simulink model "samerHARDWAREPOTread"  (R2025b)
settings: Solver=FixedStepDiscrete  StartTime=0.0  StopTime=inf  RelTol=1e-3  EnableMultiTasking=on
libraries: arduinolib x18, slpidlib x6, simulink x2
settings Model: ExtModeTrigDuration=2  Creator=Ahmed Sedky  LastModifiedBy=Samer FARAJ
settings OptimizationCC: EnhancedBackFolding=on  PassReuseOutputArgsAs=Individual arguments  ZeroExternalMemoryAtStartup=off  ZeroInternalMemoryAtStartup=off  MaxStackSize=64  OptimizeBlockOrder=speed  DifferentSizesBufferReuse=on  OptimizationCustomize=off  EfficientTunableParamExpr=on
settings DebuggingCC: ParameterTunabilityLossMsg=error
settings HardwareCC: ProdBitPerInt=16.0  ProdBitPerPointer=16.0  ProdBitPerSizeT=16.0  ProdBitPerPtrDiffT=16.0  ProdLargestAtomicFloat=None  ProdWordSize=8.0  ProdHWDeviceType=Atmel->AVR
settings SFSimCC: MATLABDynamicMemAlloc=off
settings RTWCC: SystemTargetFile=ert.tlc  HardwareBoard=Arduino Mega 2560  TemplateMakefile=ert_default_tmf  Toolchain=Arduino AVR  BuildConfiguration=Faster Runs  GPUComputeCapability=3.5  Description=Embedded Coder
settings CodeAppCC: ForceParamTrailComments=on  IgnoreCustomStorageClasses=off  OperatorAnnotations=on  SimulinkDataObjDesc=on  SFDataObjDesc=on  InsertBlockDesc=on
settings ERTTargetCC: ExtModeTransport=3.0  ExtModeStaticAlloc=on  ExtModeAutomaticAllocSize=off  ExtModeStaticAllocSize=2048.0  ExtModeMexFile=ext_xcp  ExtModeIntrfLevel=Level2 - Open  InlinedParameterPlacement=Hierarchical  DynamicArrayContainerType=coder::array  SupportContinuousTime=on  SupportVariableSizeSignals=on

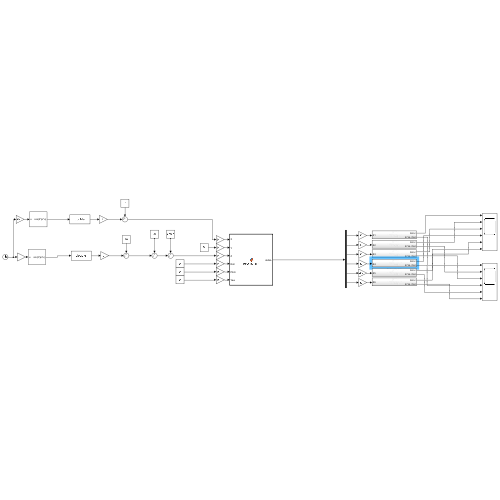
[thumbnail: Simulink's stored preview of the top-level diagram]
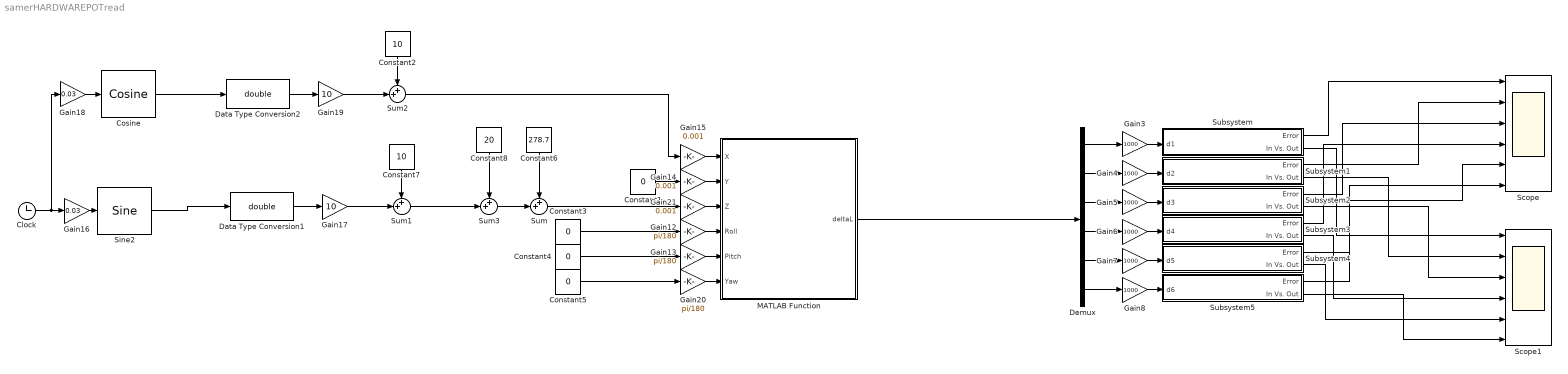
== system samerHARDWAREPOTread ==
  Clock : Clock
  Constant{1,3..5} (4 alike) : Constant  Value=0
  Constant2 : Constant  Value=10
  Constant6 : Constant  Value=278.7
  Constant7 : Constant  Value=10
  Constant8 : Constant  Value=20
  Cosine : simulink/Lookup Tables/Cosine  Formula=cos(2*pi*u)  NumDataPoints=(2^5)+1  OutputWordLength=16  InternalRulePriority=Speed
  Data Type Conversion1 : DataTypeConversion  OutDataTypeStr=double  SaturateOnIntegerOverflow=off  RndMeth=Floor
  Data Type Conversion2 : DataTypeConversion  OutDataTypeStr=double  SaturateOnIntegerOverflow=off  RndMeth=Floor
  Demux : Demux  Outputs=6
  Gain12 : Gain  Gain=pi/180
  Gain13 : Gain  Gain=pi/180
  Gain14 : Gain  Gain=0.001
  Gain15 : Gain  Gain=0.001
  Gain16 : Gain  Gain=0.03
  Gain17 : Gain  Gain=10
  Gain18 : Gain  Gain=0.03
  Gain19 : Gain  Gain=10
  Gain20 : Gain  Gain=pi/180
  Gain21 : Gain  Gain=0.001
  Gain{3..8} (6 alike) : Gain  Gain=1000
  MATLAB Function : MATLAB Function  TreatAsAtomicUnit=on
  Scope : Scope  NumInputPorts=6
      settings: ActiveDisplayYMinimum=15.51881  ActiveDisplayYMaximum=26.12546
  Scope1 : Scope  NumInputPorts=6
      settings: ActiveDisplayYMinimum=-3.1331  ActiveDisplayYMaximum=28.1979  DataLoggingVariableName=ScopeData2
  Sine2 : simulink/Lookup Tables/Sine  Formula=sin(2*pi*u)  NumDataPoints=(2^5)+1  OutputWordLength=16  InternalRulePriority=Speed
  Subsystem : Subsystem
  Subsystem1 : Subsystem
  Subsystem2 : Subsystem
  Subsystem3 : Subsystem
  Subsystem4 : Subsystem
  Subsystem5 : Subsystem
  Sum{,1..3} (4 alike) : Sum  Inputs=++|
  wires:
  Demux/1 -> Gain3/1
  Demux/6 -> Gain8/1
  Demux/3 -> Gain5/1
  Demux/4 -> Gain6/1
  Demux/5 -> Gain7/1
  Demux/2 -> Gain4/1
  Gain3/1 -> Subsystem/1(d1)
  Gain4/1 -> Subsystem1/1(d2)
  Gain5/1 -> Subsystem2/1(d3)
  Gain6/1 -> Subsystem3/1(d4)
  Gain7/1 -> Subsystem4/1(d5)
  Gain8/1 -> Subsystem5/1(d6)
  Subsystem/1(Error) -> Scope/1
  Subsystem1/1(Error) -> Scope/2
  Subsystem2/1(Error) -> Scope/3
  Subsystem3/1(Error) -> Scope/4
  Subsystem4/1(Error) -> Scope/5
  Subsystem5/1(Error) -> Scope/6
  Subsystem/2(In Vs. Out) -> Scope1/1
  Subsystem1/2(In Vs. Out) -> Scope1/2
  Subsystem2/2(In Vs. Out) -> Scope1/3
  Subsystem3/2(In Vs. Out) -> Scope1/4
  Subsystem4/2(In Vs. Out) -> Scope1/5
  Subsystem5/2(In Vs. Out) -> Scope1/6
  Constant8/1 -> Sum3/1
  Gain21/1 -> MATLAB Function/3(Z)
  Gain18/1 -> Cosine/1
  Gain15/1 -> MATLAB Function/1(X)
  Sum3/1 -> Sum/2
  Gain16/1 -> Sine2/1
  Cosine/1 -> Data Type Conversion2/1
  Gain20/1 -> MATLAB Function/6(Yaw)
  Gain19/1 -> Sum2/2
  Gain17/1 -> Sum1/2
  Data Type Conversion2/1 -> Gain19/1
  Constant6/1 -> Sum/1
  Sine2/1 -> Data Type Conversion1/1
  Constant7/1 -> Sum1/1
  Constant3/1 -> Gain12/1
  Clock/1 -> Gain16/1, Gain18/1
  Constant2/1 -> Sum2/1
  Sum/1 -> Gain21/1
  Gain14/1 -> MATLAB Function/2(Y)
  Constant1/1 -> Gain14/1
  Constant5/1 -> Gain20/1
  Sum1/1 -> Sum3/2
  Sum2/1 -> Gain15/1
  Constant4/1 -> Gain13/1
  Gain12/1 -> MATLAB Function/4(Roll)
  Data Type Conversion1/1 -> Gain17/1
  Gain13/1 -> MATLAB Function/5(Pitch)
  MATLAB Function/1(deltaL) -> Demux/1

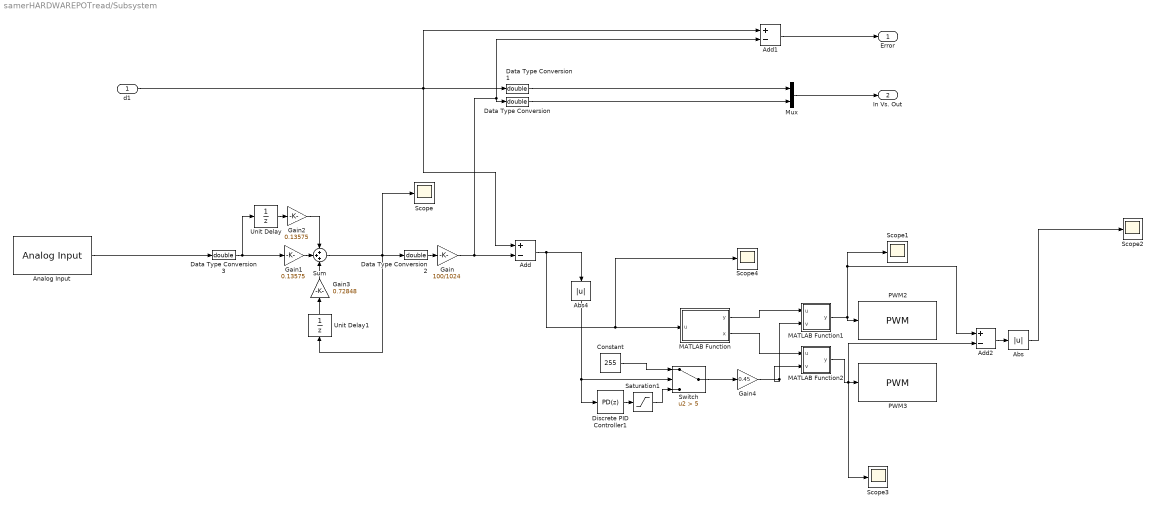
== system samerHARDWAREPOTread/Subsystem ==
  d1 : Inport
  Abs : Abs  SaturateOnIntegerOverflow=off
  Abs4 : Abs  SaturateOnIntegerOverflow=off
  Add : Sum  Inputs=+-
  Add1 : Sum  Inputs=+-
  Add2 : Sum  Inputs=+-
  Analog Input : arduinolib/Analog Input  pinNumber=0  ReadResultsOnly=off  ConversionTriggerSource=Software  ExternalTriggerType=uint32( 0 )  OutputDataType=uint16  EnableConversionCompleteNotify=off  EnableOuputStatus=off  SampleTime=0.01  blockPlatform=arduino
  Constant : Constant  Value=255
  Data Type Conversion{,1..3} (4 alike) : DataTypeConversion  OutDataTypeStr=double  SaturateOnIntegerOverflow=off  RndMeth=Floor
  Discrete PID Controller1 : slpidlib/PID Controller  Controller=PD  Form=Parallel  TimeDomain=Discrete-time  UseExternalTs=off  SampleTime=0.01  IntegratorMethod=Forward Euler  FilterMethod=Forward Euler  ControllerParametersSource=internal  P=325  I=3  UseKiTs=off  D=.75  UseExternalDerivativeSource=off  N=1  UseFilter=off  TunerSelectOption=Transfer Function Based (PID Tuner App)  InitialConditionSource=internal  InitialConditionForIntegrator=0  InitialConditionForFilter=0  DifferentiatorICPrevScaledInput=0  ExternalReset=none  TrackingMode=off  Kt=1  LimitOutput=off  SatLimitsSource=internal  UpperSaturationLimit=inf  LowerSaturationLimit=-inf  LinearizeAsGain=off  AntiWindupMode=none  Kb=1  LimitIntegrator=off  UpperIntegratorSaturationLimit=inf  LowerIntegratorSaturationLimit=-inf  POutMin=[]  POutMax=[]  IOutMin=[]  IOutMax=[]  DOutMin=[]  DOutMax=[]  NOutMin=[]  NOutMax=[]  SumOutMin=[]  SumOutMax=[]  SaturationOutMin=[]  SaturationOutMax=[]  PParamMin=[]  PParamMax=[]  IParamMin=[]  IParamMax=[]  DParamMin=[]  DParamMax=[]  NParamMin=[]  NParamMax=[]  KbParamMin=[]  KbParamMax=[]  KtParamMin=[]  KtParamMax=[]  KbOutMin=[]  KbOutMax=[]  KtOutMin=[]  KtOutMax=[]  IntegratorOutMin=[]  IntegratorOutMax=[]  FilterOutMin=[]  FilterOutMax=[]  SumI1OutMin=[]  SumI1OutMax=[]  SumI2OutMin=[]  SumI2OutMax=[]  SumI3OutMin=[]  SumI3OutMax=[]  SumI4OutMin=[]  SumI4OutMax=[]  SumDOutMin=[]  SumDOutMax=[]  DifferentiatorOutMin=[]  DifferentiatorOutMax=[]  FilterDiffOutCoefMin=[]  FilterDiffOutCoefMax=[]  ReciprocalOutMin=[]  ReciprocalOutMax=[]  SumDenOutMin=[]  SumDenOutMax=[]  SumNumOutMin=[]  SumNumOutMax=[]  DivideOutMin=[]  DivideOutMax=[]  UdiffTsProdOutMin=[]  UdiffTsProdOutMax=[]  NTsProdOutMin=[]  NTsProdOutMax=[]  UintegralTsProdOutMin=[]  UintegralTsProdOutMax=[]  UngainTsProdOutMin=[]  UngainTsProdOutMax=[]  ClampingZeroOutDataTypeStr=Inherit: Inherit via back propagation  ClampingZeroOutMin=[]  ClampingZeroOutMax=[]  FilterDenConstantOutDataTypeStr=Inherit: Inherit via back propagation  FilterDenConstantOutMin=[]  FilterDenConstantOutMax=[]  PCopyOutDataTypeStr=Inherit: Inherit via back propagation  PCopyOutMin=[]  PCopyOutMax=[]  NCopyOutDataTypeStr=Inherit: Inherit via back propagation  NCopyOutMin=[]  NCopyOutMax=[]  IntegratorContinuousStateAttributes=''  IntegratorStateMustResolveToSignalObject=off  IntegratorRTWStateStorageClass=Auto  FilterContinuousStateAttributes=''  FilterStateMustResolveToSignalObject=off  FilterRTWStateStorageClass=Auto  ParallelPVariant=InternalParameters  IdealPVariant=Disabled  IVariant=Disabled  DVariant=InternalParameters  IntegratorVariant=Disabled  SatVariant=Disabled  AWVariant=Disabled  PCopyVariant=Disabled  TRVariant=Disabled  FdbkBlocksVariant=Forward  IdealPFdbkVariant=Disabled  SatFdbkVariant=Disabled  DerivativeFilterVariant=Differentiator  NVariant=Passthrough  NCopyVariant=Disabled_SignalSpec  FilterICVariant=InternalICsDifferentiator  IntegratorICVariant=Disabled  ExternalResetVariant=Disabled  TRSumVariant=Passthrough  SumFdbkVariant=Disabled  SumVariant=Sum_PD  TsampFilterVariant=InternalTs  TsampNgainVariant=Passthrough  TsampIntegralVariant=Disabled_SignalSpec  ExternalSaturationOutDataTypeStr=Inherit: Same as second input  DerivativeSourceVariant=ErrorSignal  PreIntVariant=InternalPreInt
      settings: LibrarySourceBlock=simulink/Discrete/Discrete PID Controller
  Gain : Gain  Gain=100/1024
  Gain1 : Gain  Gain=0.13575
  Gain2 : Gain  Gain=0.13575
  Gain3 : Gain  Gain=0.72848
  Gain4 : Gain  Gain=0.45
  MATLAB Function : MATLAB Function  TreatAsAtomicUnit=on
  MATLAB Function1 : MATLAB Function  TreatAsAtomicUnit=on
  MATLAB Function2 : MATLAB Function  TreatAsAtomicUnit=on
  Mux : Mux  Inputs=2
  PWM2 : arduinolib/PWM  pinNumber=2  frequencyType=Default  desiredFrequency=490.2  achievableFrequency=490.2
  PWM3 : arduinolib/PWM  pinNumber=3  frequencyType=Default  desiredFrequency=490.2  achievableFrequency=490.2
  Saturation1 : Saturate  UpperLimit=200  LowerLimit=0
  Scope{,1..4} (5 alike) : Scope
      Scope settings: ActiveDisplayYMinimum=-89.3058  ActiveDisplayYMaximum=803.75221
      Scope1 settings: ActiveDisplayYMinimum=-31.875  ActiveDisplayYMaximum=286.875  DataLoggingVariableName=ScopeData2
      Scope2 settings: DataLoggingVariableName=ScopeData3
      Scope3 settings: ActiveDisplayYMinimum=-31.875  ActiveDisplayYMaximum=286.875  DataLoggingVariableName=ScopeData4
      Scope4 settings: ActiveDisplayYMinimum=-38.33565  ActiveDisplayYMaximum=48.7182
  Sum : Sum  Inputs=+++
  Switch : Switch  Criteria=u2 > Threshold  Threshold=5  SaturateOnIntegerOverflow=off  InputSameDT=off
  Unit Delay : UnitDelay  SampleTime=-1  HasFrameUpgradeWarning=on
  Unit Delay1 : UnitDelay  SampleTime=-1  HasFrameUpgradeWarning=on
  Error : Outport
  In Vs. Out : Outport  Port=2
  wires:
  Unit Delay/1 -> Gain2/1
  Gain3/1 -> Sum/3
  Add2/1 -> Abs/1
  MATLAB Function1/1(y) -> PWM2/1, Add2/1, Scope1/1
  Data Type Conversion2/1 -> Gain/1
  Abs/1 -> Scope2/1
  MATLAB Function2/1(y) -> Scope3/1, Add2/2, PWM3/1
  Add/1 -> Abs4/1, Scope4/1, MATLAB Function/1(u)
  Saturation1/1 -> Switch/3
  Analog Input/1 -> Data Type Conversion3/1
  Unit Delay1/1 -> Gain3/1
  Gain/1 -> Data Type Conversion/1, Add1/2, Add/2
  d1/1 -> Data Type Conversion1/1, Add1/1, Add/1
  Discrete PID Controller1/1 -> Saturation1/1
  Constant/1 -> Switch/1
  Data Type Conversion/1 -> Mux/2
  Data Type Conversion1/1 -> Mux/1
  Mux/1 -> In Vs. Out/1
  Data Type Conversion3/1 -> Unit Delay/1, Gain1/1
  Sum/1 -> Scope/1, Data Type Conversion2/1, Unit Delay1/1
  Abs4/1 -> Discrete PID Controller1/1, Switch/2
  Switch/1 -> Gain4/1
  Gain4/1 -> MATLAB Function2/2(v), MATLAB Function1/2(v)
  MATLAB Function/1(y) -> MATLAB Function1/1(u)
  MATLAB Function/2(x) -> MATLAB Function2/1(u)
  Gain1/1 -> Sum/2
  Gain2/1 -> Sum/1
  Add1/1 -> Error/1

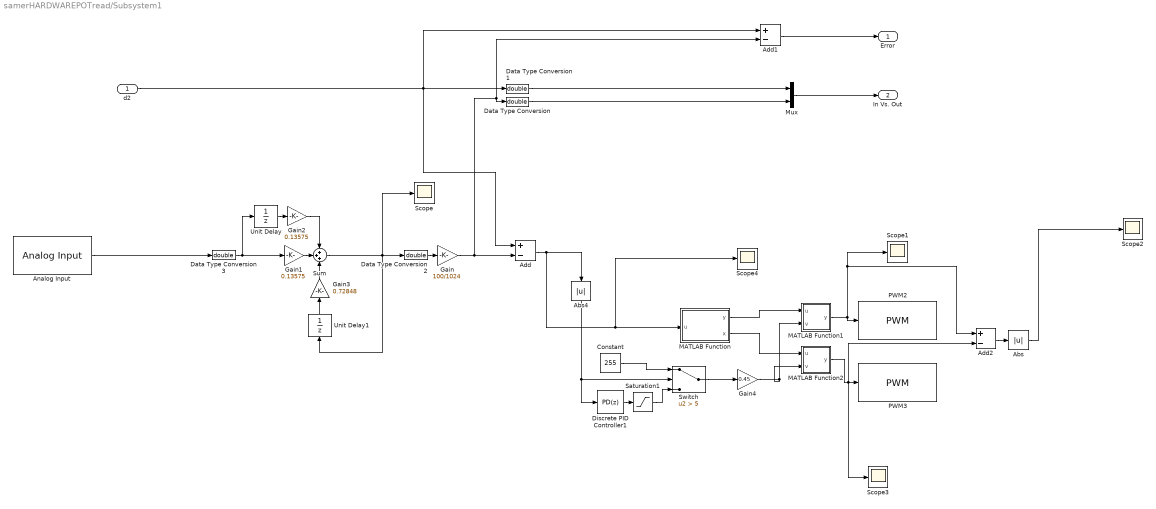
== system samerHARDWAREPOTread/Subsystem1 ==
  d2 : Inport
  Abs : Abs  SaturateOnIntegerOverflow=off
  Abs4 : Abs  SaturateOnIntegerOverflow=off
  Add : Sum  Inputs=+-
  Add1 : Sum  Inputs=+-
  Add2 : Sum  Inputs=+-
  Analog Input : arduinolib/Analog Input  pinNumber=5  ReadResultsOnly=off  ConversionTriggerSource=Software  ExternalTriggerType=uint32( 0 )  OutputDataType=uint16  EnableConversionCompleteNotify=off  EnableOuputStatus=off  SampleTime=0.01  blockPlatform=arduino
  Constant : Constant  Value=255
  Data Type Conversion{,1..3} (4 alike) : DataTypeConversion  OutDataTypeStr=double  SaturateOnIntegerOverflow=off  RndMeth=Floor
  Discrete PID Controller1 : slpidlib/PID Controller  Controller=PD  Form=Parallel  TimeDomain=Discrete-time  UseExternalTs=off  SampleTime=0.01  IntegratorMethod=Forward Euler  FilterMethod=Forward Euler  ControllerParametersSource=internal  P=325  I=3  UseKiTs=off  D=.75  N=1  UseFilter=off  TunerSelectOption=Transfer Function Based (PID Tuner App)  InitialConditionSource=internal  InitialConditionForIntegrator=0  InitialConditionForFilter=0  DifferentiatorICPrevScaledInput=0  ExternalReset=none  TrackingMode=off  Kt=1  LimitOutput=off  SatLimitsSource=internal  UpperSaturationLimit=inf  LowerSaturationLimit=-inf  LinearizeAsGain=off  AntiWindupMode=none  Kb=1  LimitIntegrator=off  UpperIntegratorSaturationLimit=inf  LowerIntegratorSaturationLimit=-inf  POutMin=[]  POutMax=[]  IOutMin=[]  IOutMax=[]  DOutMin=[]  DOutMax=[]  NOutMin=[]  NOutMax=[]  SumOutMin=[]  SumOutMax=[]  SaturationOutMin=[]  SaturationOutMax=[]  PParamMin=[]  PParamMax=[]  IParamMin=[]  IParamMax=[]  DParamMin=[]  DParamMax=[]  NParamMin=[]  NParamMax=[]  KbParamMin=[]  KbParamMax=[]  KtParamMin=[]  KtParamMax=[]  KbOutMin=[]  KbOutMax=[]  KtOutMin=[]  KtOutMax=[]  IntegratorOutMin=[]  IntegratorOutMax=[]  FilterOutMin=[]  FilterOutMax=[]  SumI1OutMin=[]  SumI1OutMax=[]  SumI2OutMin=[]  SumI2OutMax=[]  SumI3OutMin=[]  SumI3OutMax=[]  SumI4OutMin=[]  SumI4OutMax=[]  SumDOutMin=[]  SumDOutMax=[]  DifferentiatorOutMin=[]  DifferentiatorOutMax=[]  FilterDiffOutCoefMin=[]  FilterDiffOutCoefMax=[]  ReciprocalOutMin=[]  ReciprocalOutMax=[]  SumDenOutMin=[]  SumDenOutMax=[]  SumNumOutMin=[]  SumNumOutMax=[]  DivideOutMin=[]  DivideOutMax=[]  UdiffTsProdOutMin=[]  UdiffTsProdOutMax=[]  NTsProdOutMin=[]  NTsProdOutMax=[]  UintegralTsProdOutMin=[]  UintegralTsProdOutMax=[]  UngainTsProdOutMin=[]  UngainTsProdOutMax=[]  ClampingZeroOutDataTypeStr=Inherit: Inherit via back propagation  ClampingZeroOutMin=[]  ClampingZeroOutMax=[]  FilterDenConstantOutDataTypeStr=Inherit: Inherit via back propagation  FilterDenConstantOutMin=[]  FilterDenConstantOutMax=[]  PCopyOutDataTypeStr=Inherit: Inherit via back propagation  PCopyOutMin=[]  PCopyOutMax=[]  NCopyOutDataTypeStr=Inherit: Inherit via back propagation  NCopyOutMin=[]  NCopyOutMax=[]  IntegratorContinuousStateAttributes=''  IntegratorStateMustResolveToSignalObject=off  IntegratorRTWStateStorageClass=Auto  FilterContinuousStateAttributes=''  FilterStateMustResolveToSignalObject=off  FilterRTWStateStorageClass=Auto  ParallelPVariant=InternalParameters  IdealPVariant=Disabled  IVariant=Disabled  DVariant=InternalParameters  IntegratorVariant=Disabled  SatVariant=Disabled  AWVariant=Disabled  PCopyVariant=Disabled  TRVariant=Disabled  FdbkBlocksVariant=Forward  IdealPFdbkVariant=Disabled  SatFdbkVariant=Disabled  DerivativeFilterVariant=Differentiator  NVariant=Passthrough  NCopyVariant=Disabled_SignalSpec  FilterICVariant=InternalICsDifferentiator  IntegratorICVariant=Disabled  ExternalResetVariant=Disabled  TRSumVariant=Passthrough  SumFdbkVariant=Disabled  SumVariant=Sum_PD  TsampFilterVariant=InternalTs  TsampNgainVariant=Passthrough  TsampIntegralVariant=Disabled_SignalSpec  ExternalSaturationOutDataTypeStr=Inherit: Same as second input
      settings: LibrarySourceBlock=simulink/Discrete/Discrete PID Controller
  Gain : Gain  Gain=100/1024
  Gain1 : Gain  Gain=0.13575
  Gain2 : Gain  Gain=0.13575
  Gain3 : Gain  Gain=0.72848
  Gain4 : Gain  Gain=0.45
  MATLAB Function : MATLAB Function  TreatAsAtomicUnit=on
  MATLAB Function1 : MATLAB Function  TreatAsAtomicUnit=on
  MATLAB Function2 : MATLAB Function  TreatAsAtomicUnit=on
  Mux : Mux  Inputs=2
  PWM2 : arduinolib/PWM  pinNumber=4  frequencyType=Default  desiredFrequency=490.2  achievableFrequency=490.2
  PWM3 : arduinolib/PWM  pinNumber=5  frequencyType=Default  desiredFrequency=490.2  achievableFrequency=490.2
  Saturation1 : Saturate  UpperLimit=200  LowerLimit=0
  Scope{,1..4} (5 alike) : Scope
      Scope settings: ActiveDisplayYMinimum=-89.3058  ActiveDisplayYMaximum=803.75221
      Scope1 settings: ActiveDisplayYMinimum=-31.875  ActiveDisplayYMaximum=286.875  DataLoggingVariableName=ScopeData2
      Scope2 settings: DataLoggingVariableName=ScopeData3
      Scope3 settings: ActiveDisplayYMinimum=-31.875  ActiveDisplayYMaximum=286.875  DataLoggingVariableName=ScopeData4
      Scope4 settings: ActiveDisplayYMinimum=-38.33565  ActiveDisplayYMaximum=48.7182
  Sum : Sum  Inputs=+++
  Switch : Switch  Criteria=u2 > Threshold  Threshold=5  SaturateOnIntegerOverflow=off  InputSameDT=off
  Unit Delay : UnitDelay  SampleTime=-1  HasFrameUpgradeWarning=on
  Unit Delay1 : UnitDelay  SampleTime=-1  HasFrameUpgradeWarning=on
  Error : Outport
  In Vs. Out : Outport  Port=2
  wires:
  Unit Delay/1 -> Gain2/1
  Gain3/1 -> Sum/3
  Add2/1 -> Abs/1
  MATLAB Function1/1(y) -> PWM2/1, Add2/1, Scope1/1
  Data Type Conversion2/1 -> Gain/1
  Abs/1 -> Scope2/1
  MATLAB Function2/1(y) -> Scope3/1, Add2/2, PWM3/1
  Add/1 -> Abs4/1, Scope4/1, MATLAB Function/1(u)
  Saturation1/1 -> Switch/3
  Analog Input/1 -> Data Type Conversion3/1
  Unit Delay1/1 -> Gain3/1
  Gain/1 -> Data Type Conversion/1, Add1/2, Add/2
  d2/1 -> Data Type Conversion1/1, Add1/1, Add/1
  Discrete PID Controller1/1 -> Saturation1/1
  Constant/1 -> Switch/1
  Data Type Conversion/1 -> Mux/2
  Data Type Conversion1/1 -> Mux/1
  Mux/1 -> In Vs. Out/1
  Data Type Conversion3/1 -> Unit Delay/1, Gain1/1
  Sum/1 -> Scope/1, Data Type Conversion2/1, Unit Delay1/1
  Abs4/1 -> Discrete PID Controller1/1, Switch/2
  Switch/1 -> Gain4/1
  Gain4/1 -> MATLAB Function2/2(v), MATLAB Function1/2(v)
  MATLAB Function/1(y) -> MATLAB Function1/1(u)
  MATLAB Function/2(x) -> MATLAB Function2/1(u)
  Gain1/1 -> Sum/2
  Gain2/1 -> Sum/1
  Add1/1 -> Error/1

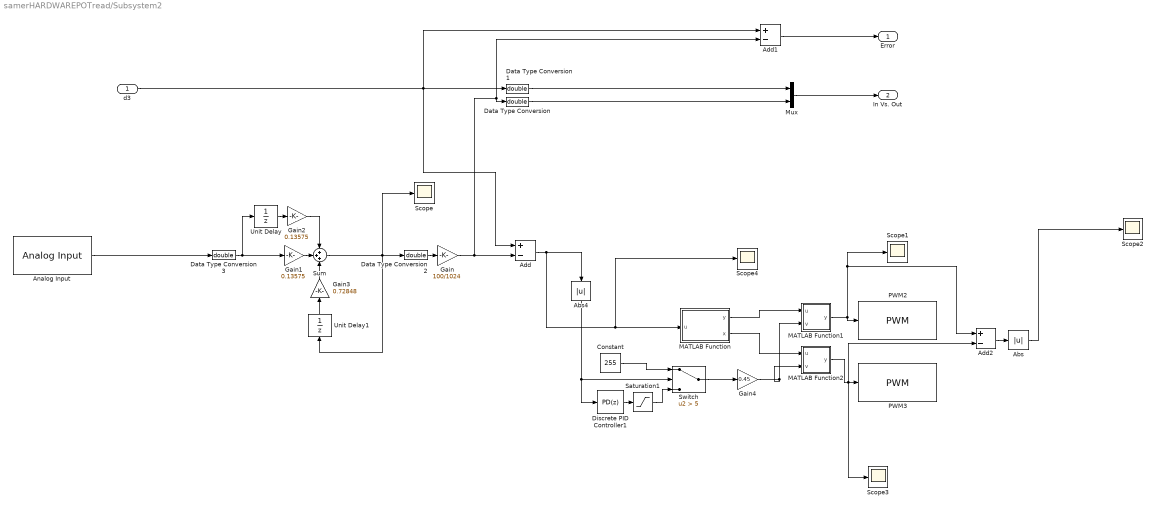
== system samerHARDWAREPOTread/Subsystem2 ==
  d3 : Inport
  Abs : Abs  SaturateOnIntegerOverflow=off
  Abs4 : Abs  SaturateOnIntegerOverflow=off
  Add : Sum  Inputs=+-
  Add1 : Sum  Inputs=+-
  Add2 : Sum  Inputs=+-
  Analog Input : arduinolib/Analog Input  pinNumber=4  ReadResultsOnly=off  ConversionTriggerSource=Software  ExternalTriggerType=uint32( 0 )  OutputDataType=uint16  EnableConversionCompleteNotify=off  EnableOuputStatus=off  SampleTime=0.01  blockPlatform=arduino
  Constant : Constant  Value=255
  Data Type Conversion{,1..3} (4 alike) : DataTypeConversion  OutDataTypeStr=double  SaturateOnIntegerOverflow=off  RndMeth=Floor
  Discrete PID Controller1 : slpidlib/PID Controller  Controller=PD  Form=Parallel  TimeDomain=Discrete-time  UseExternalTs=off  SampleTime=0.01  IntegratorMethod=Forward Euler  FilterMethod=Forward Euler  ControllerParametersSource=internal  P=325  I=3  UseKiTs=off  D=.75  UseExternalDerivativeSource=off  N=1  UseFilter=off  TunerSelectOption=Transfer Function Based (PID Tuner App)  InitialConditionSource=internal  InitialConditionForIntegrator=0  InitialConditionForFilter=0  DifferentiatorICPrevScaledInput=0  ExternalReset=none  TrackingMode=off  Kt=1  LimitOutput=off  SatLimitsSource=internal  UpperSaturationLimit=inf  LowerSaturationLimit=-inf  LinearizeAsGain=off  AntiWindupMode=none  Kb=1  LimitIntegrator=off  UpperIntegratorSaturationLimit=inf  LowerIntegratorSaturationLimit=-inf  POutMin=[]  POutMax=[]  IOutMin=[]  IOutMax=[]  DOutMin=[]  DOutMax=[]  NOutMin=[]  NOutMax=[]  SumOutMin=[]  SumOutMax=[]  SaturationOutMin=[]  SaturationOutMax=[]  PParamMin=[]  PParamMax=[]  IParamMin=[]  IParamMax=[]  DParamMin=[]  DParamMax=[]  NParamMin=[]  NParamMax=[]  KbParamMin=[]  KbParamMax=[]  KtParamMin=[]  KtParamMax=[]  KbOutMin=[]  KbOutMax=[]  KtOutMin=[]  KtOutMax=[]  IntegratorOutMin=[]  IntegratorOutMax=[]  FilterOutMin=[]  FilterOutMax=[]  SumI1OutMin=[]  SumI1OutMax=[]  SumI2OutMin=[]  SumI2OutMax=[]  SumI3OutMin=[]  SumI3OutMax=[]  SumI4OutMin=[]  SumI4OutMax=[]  SumDOutMin=[]  SumDOutMax=[]  DifferentiatorOutMin=[]  DifferentiatorOutMax=[]  FilterDiffOutCoefMin=[]  FilterDiffOutCoefMax=[]  ReciprocalOutMin=[]  ReciprocalOutMax=[]  SumDenOutMin=[]  SumDenOutMax=[]  SumNumOutMin=[]  SumNumOutMax=[]  DivideOutMin=[]  DivideOutMax=[]  UdiffTsProdOutMin=[]  UdiffTsProdOutMax=[]  NTsProdOutMin=[]  NTsProdOutMax=[]  UintegralTsProdOutMin=[]  UintegralTsProdOutMax=[]  UngainTsProdOutMin=[]  UngainTsProdOutMax=[]  ClampingZeroOutDataTypeStr=Inherit: Inherit via back propagation  ClampingZeroOutMin=[]  ClampingZeroOutMax=[]  FilterDenConstantOutDataTypeStr=Inherit: Inherit via back propagation  FilterDenConstantOutMin=[]  FilterDenConstantOutMax=[]  PCopyOutDataTypeStr=Inherit: Inherit via back propagation  PCopyOutMin=[]  PCopyOutMax=[]  NCopyOutDataTypeStr=Inherit: Inherit via back propagation  NCopyOutMin=[]  NCopyOutMax=[]  IntegratorContinuousStateAttributes=''  IntegratorStateMustResolveToSignalObject=off  IntegratorRTWStateStorageClass=Auto  FilterContinuousStateAttributes=''  FilterStateMustResolveToSignalObject=off  FilterRTWStateStorageClass=Auto  ParallelPVariant=InternalParameters  IdealPVariant=Disabled  IVariant=Disabled  DVariant=InternalParameters  IntegratorVariant=Disabled  SatVariant=Disabled  AWVariant=Disabled  PCopyVariant=Disabled  TRVariant=Disabled  FdbkBlocksVariant=Forward  IdealPFdbkVariant=Disabled  SatFdbkVariant=Disabled  DerivativeFilterVariant=Differentiator  NVariant=Passthrough  NCopyVariant=Disabled_SignalSpec  FilterICVariant=InternalICsDifferentiator  IntegratorICVariant=Disabled  ExternalResetVariant=Disabled  TRSumVariant=Passthrough  SumFdbkVariant=Disabled  SumVariant=Sum_PD  TsampFilterVariant=InternalTs  TsampNgainVariant=Passthrough  TsampIntegralVariant=Disabled_SignalSpec  ExternalSaturationOutDataTypeStr=Inherit: Same as second input  DerivativeSourceVariant=ErrorSignal  PreIntVariant=InternalPreInt
      settings: LibrarySourceBlock=simulink/Discrete/Discrete PID Controller
  Gain : Gain  Gain=100/1024
  Gain1 : Gain  Gain=0.13575
  Gain2 : Gain  Gain=0.13575
  Gain3 : Gain  Gain=0.72848
  Gain4 : Gain  Gain=0.45
  MATLAB Function : MATLAB Function  TreatAsAtomicUnit=on
  MATLAB Function1 : MATLAB Function  TreatAsAtomicUnit=on
  MATLAB Function2 : MATLAB Function  TreatAsAtomicUnit=on
  Mux : Mux  Inputs=2
  PWM2 : arduinolib/PWM  pinNumber=10  frequencyType=Default  desiredFrequency=490.2  achievableFrequency=490.2
  PWM3 : arduinolib/PWM  pinNumber=11  frequencyType=Default  desiredFrequency=490.2  achievableFrequency=490.2
  Saturation1 : Saturate  UpperLimit=200  LowerLimit=0
  Scope{,1..4} (5 alike) : Scope
      Scope settings: ActiveDisplayYMinimum=-89.3058  ActiveDisplayYMaximum=803.75221
      Scope1 settings: ActiveDisplayYMinimum=-31.875  ActiveDisplayYMaximum=286.875  DataLoggingVariableName=ScopeData2
      Scope2 settings: DataLoggingVariableName=ScopeData3
      Scope3 settings: ActiveDisplayYMinimum=-31.875  ActiveDisplayYMaximum=286.875  DataLoggingVariableName=ScopeData4
      Scope4 settings: ActiveDisplayYMinimum=-38.33565  ActiveDisplayYMaximum=48.7182
  Sum : Sum  Inputs=+++
  Switch : Switch  Criteria=u2 > Threshold  Threshold=5  SaturateOnIntegerOverflow=off  InputSameDT=off
  Unit Delay : UnitDelay  SampleTime=-1  HasFrameUpgradeWarning=on
  Unit Delay1 : UnitDelay  SampleTime=-1  HasFrameUpgradeWarning=on
  Error : Outport
  In Vs. Out : Outport  Port=2
  wires:
  Unit Delay/1 -> Gain2/1
  Gain3/1 -> Sum/3
  Add2/1 -> Abs/1
  MATLAB Function1/1(y) -> PWM2/1, Add2/1, Scope1/1
  Data Type Conversion2/1 -> Gain/1
  Abs/1 -> Scope2/1
  MATLAB Function2/1(y) -> Scope3/1, Add2/2, PWM3/1
  Add/1 -> Abs4/1, Scope4/1, MATLAB Function/1(u)
  Saturation1/1 -> Switch/3
  Analog Input/1 -> Data Type Conversion3/1
  Unit Delay1/1 -> Gain3/1
  Gain/1 -> Data Type Conversion/1, Add1/2, Add/2
  d3/1 -> Data Type Conversion1/1, Add1/1, Add/1
  Discrete PID Controller1/1 -> Saturation1/1
  Constant/1 -> Switch/1
  Data Type Conversion/1 -> Mux/2
  Data Type Conversion1/1 -> Mux/1
  Mux/1 -> In Vs. Out/1
  Data Type Conversion3/1 -> Unit Delay/1, Gain1/1
  Sum/1 -> Scope/1, Data Type Conversion2/1, Unit Delay1/1
  Abs4/1 -> Discrete PID Controller1/1, Switch/2
  Switch/1 -> Gain4/1
  Gain4/1 -> MATLAB Function2/2(v), MATLAB Function1/2(v)
  MATLAB Function/1(y) -> MATLAB Function1/1(u)
  MATLAB Function/2(x) -> MATLAB Function2/1(u)
  Gain1/1 -> Sum/2
  Gain2/1 -> Sum/1
  Add1/1 -> Error/1

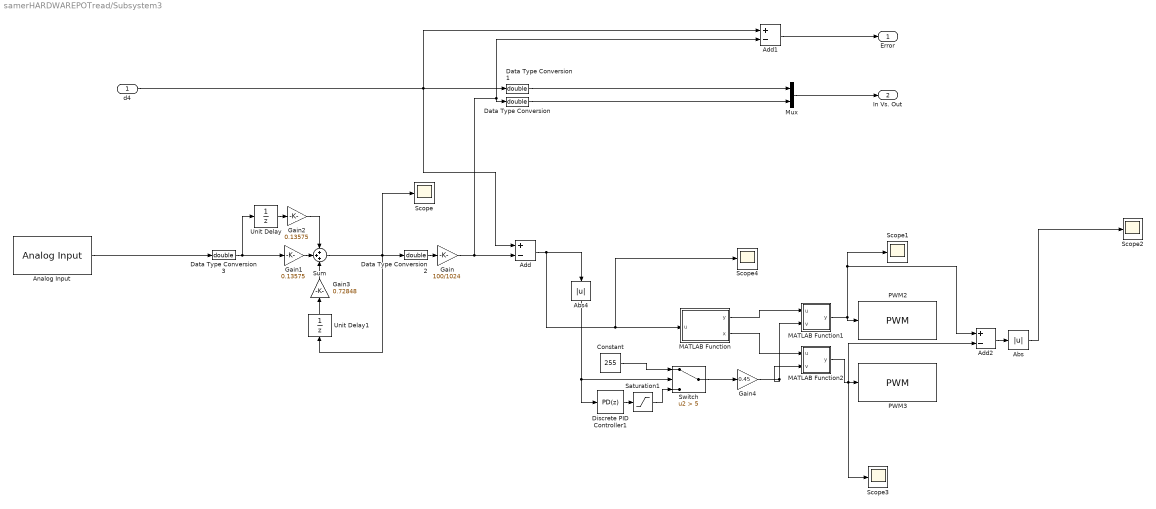
== system samerHARDWAREPOTread/Subsystem3 ==
  d4 : Inport
  Abs : Abs  SaturateOnIntegerOverflow=off
  Abs4 : Abs  SaturateOnIntegerOverflow=off
  Add : Sum  Inputs=+-
  Add1 : Sum  Inputs=+-
  Add2 : Sum  Inputs=+-
  Analog Input : arduinolib/Analog Input  pinNumber=3  ReadResultsOnly=off  ConversionTriggerSource=Software  ExternalTriggerType=uint32( 0 )  OutputDataType=uint16  EnableConversionCompleteNotify=off  EnableOuputStatus=off  SampleTime=0.01  blockPlatform=arduino
  Constant : Constant  Value=255
  Data Type Conversion{,1..3} (4 alike) : DataTypeConversion  OutDataTypeStr=double  SaturateOnIntegerOverflow=off  RndMeth=Floor
  Discrete PID Controller1 : slpidlib/PID Controller  Controller=PD  Form=Parallel  TimeDomain=Discrete-time  UseExternalTs=off  SampleTime=0.01  IntegratorMethod=Forward Euler  FilterMethod=Forward Euler  ControllerParametersSource=internal  P=325  I=3  UseKiTs=off  D=.75  UseExternalDerivativeSource=off  N=1  UseFilter=off  TunerSelectOption=Transfer Function Based (PID Tuner App)  InitialConditionSource=internal  InitialConditionForIntegrator=0  InitialConditionForFilter=0  DifferentiatorICPrevScaledInput=0  ExternalReset=none  TrackingMode=off  Kt=1  LimitOutput=off  SatLimitsSource=internal  UpperSaturationLimit=inf  LowerSaturationLimit=-inf  LinearizeAsGain=off  AntiWindupMode=none  Kb=1  LimitIntegrator=off  UpperIntegratorSaturationLimit=inf  LowerIntegratorSaturationLimit=-inf  POutMin=[]  POutMax=[]  IOutMin=[]  IOutMax=[]  DOutMin=[]  DOutMax=[]  NOutMin=[]  NOutMax=[]  SumOutMin=[]  SumOutMax=[]  SaturationOutMin=[]  SaturationOutMax=[]  PParamMin=[]  PParamMax=[]  IParamMin=[]  IParamMax=[]  DParamMin=[]  DParamMax=[]  NParamMin=[]  NParamMax=[]  KbParamMin=[]  KbParamMax=[]  KtParamMin=[]  KtParamMax=[]  KbOutMin=[]  KbOutMax=[]  KtOutMin=[]  KtOutMax=[]  IntegratorOutMin=[]  IntegratorOutMax=[]  FilterOutMin=[]  FilterOutMax=[]  SumI1OutMin=[]  SumI1OutMax=[]  SumI2OutMin=[]  SumI2OutMax=[]  SumI3OutMin=[]  SumI3OutMax=[]  SumI4OutMin=[]  SumI4OutMax=[]  SumDOutMin=[]  SumDOutMax=[]  DifferentiatorOutMin=[]  DifferentiatorOutMax=[]  FilterDiffOutCoefMin=[]  FilterDiffOutCoefMax=[]  ReciprocalOutMin=[]  ReciprocalOutMax=[]  SumDenOutMin=[]  SumDenOutMax=[]  SumNumOutMin=[]  SumNumOutMax=[]  DivideOutMin=[]  DivideOutMax=[]  UdiffTsProdOutMin=[]  UdiffTsProdOutMax=[]  NTsProdOutMin=[]  NTsProdOutMax=[]  UintegralTsProdOutMin=[]  UintegralTsProdOutMax=[]  UngainTsProdOutMin=[]  UngainTsProdOutMax=[]  ClampingZeroOutDataTypeStr=Inherit: Inherit via back propagation  ClampingZeroOutMin=[]  ClampingZeroOutMax=[]  FilterDenConstantOutDataTypeStr=Inherit: Inherit via back propagation  FilterDenConstantOutMin=[]  FilterDenConstantOutMax=[]  PCopyOutDataTypeStr=Inherit: Inherit via back propagation  PCopyOutMin=[]  PCopyOutMax=[]  NCopyOutDataTypeStr=Inherit: Inherit via back propagation  NCopyOutMin=[]  NCopyOutMax=[]  IntegratorContinuousStateAttributes=''  IntegratorStateMustResolveToSignalObject=off  IntegratorRTWStateStorageClass=Auto  FilterContinuousStateAttributes=''  FilterStateMustResolveToSignalObject=off  FilterRTWStateStorageClass=Auto  ParallelPVariant=InternalParameters  IdealPVariant=Disabled  IVariant=Disabled  DVariant=InternalParameters  IntegratorVariant=Disabled  SatVariant=Disabled  AWVariant=Disabled  PCopyVariant=Disabled  TRVariant=Disabled  FdbkBlocksVariant=Forward  IdealPFdbkVariant=Disabled  SatFdbkVariant=Disabled  DerivativeFilterVariant=Differentiator  NVariant=Passthrough  NCopyVariant=Disabled_SignalSpec  FilterICVariant=InternalICsDifferentiator  IntegratorICVariant=Disabled  ExternalResetVariant=Disabled  TRSumVariant=Passthrough  SumFdbkVariant=Disabled  SumVariant=Sum_PD  TsampFilterVariant=InternalTs  TsampNgainVariant=Passthrough  TsampIntegralVariant=Disabled_SignalSpec  ExternalSaturationOutDataTypeStr=Inherit: Same as second input  DerivativeSourceVariant=ErrorSignal  PreIntVariant=InternalPreInt
      settings: LibrarySourceBlock=simulink/Discrete/Discrete PID Controller
  Gain : Gain  Gain=100/1024
  Gain1 : Gain  Gain=0.13575
  Gain2 : Gain  Gain=0.13575
  Gain3 : Gain  Gain=0.72848
  Gain4 : Gain  Gain=0.45
  MATLAB Function : MATLAB Function  TreatAsAtomicUnit=on
  MATLAB Function1 : MATLAB Function  TreatAsAtomicUnit=on
  MATLAB Function2 : MATLAB Function  TreatAsAtomicUnit=on
  Mux : Mux  Inputs=2
  PWM2 : arduinolib/PWM  pinNumber=12  frequencyType=Default  desiredFrequency=490.2  achievableFrequency=490.2
  PWM3 : arduinolib/PWM  pinNumber=13  frequencyType=Default  desiredFrequency=490.2  achievableFrequency=490.2
  Saturation1 : Saturate  UpperLimit=200  LowerLimit=0
  Scope{,1..4} (5 alike) : Scope
      Scope settings: ActiveDisplayYMinimum=-89.3058  ActiveDisplayYMaximum=803.75221
      Scope1 settings: ActiveDisplayYMinimum=-31.875  ActiveDisplayYMaximum=286.875  DataLoggingVariableName=ScopeData2
      Scope2 settings: DataLoggingVariableName=ScopeData3
      Scope3 settings: ActiveDisplayYMinimum=-31.875  ActiveDisplayYMaximum=286.875  DataLoggingVariableName=ScopeData4
      Scope4 settings: ActiveDisplayYMinimum=-38.33565  ActiveDisplayYMaximum=48.7182
  Sum : Sum  Inputs=+++
  Switch : Switch  Criteria=u2 > Threshold  Threshold=5  SaturateOnIntegerOverflow=off  InputSameDT=off
  Unit Delay : UnitDelay  SampleTime=-1  HasFrameUpgradeWarning=on
  Unit Delay1 : UnitDelay  SampleTime=-1  HasFrameUpgradeWarning=on
  Error : Outport
  In Vs. Out : Outport  Port=2
  wires:
  Unit Delay/1 -> Gain2/1
  Gain3/1 -> Sum/3
  Add2/1 -> Abs/1
  MATLAB Function1/1(y) -> PWM2/1, Add2/1, Scope1/1
  Data Type Conversion2/1 -> Gain/1
  Abs/1 -> Scope2/1
  MATLAB Function2/1(y) -> Scope3/1, Add2/2, PWM3/1
  Add/1 -> Abs4/1, Scope4/1, MATLAB Function/1(u)
  Saturation1/1 -> Switch/3
  Analog Input/1 -> Data Type Conversion3/1
  Unit Delay1/1 -> Gain3/1
  Gain/1 -> Data Type Conversion/1, Add1/2, Add/2
  d4/1 -> Data Type Conversion1/1, Add1/1, Add/1
  Discrete PID Controller1/1 -> Saturation1/1
  Constant/1 -> Switch/1
  Data Type Conversion/1 -> Mux/2
  Data Type Conversion1/1 -> Mux/1
  Mux/1 -> In Vs. Out/1
  Data Type Conversion3/1 -> Unit Delay/1, Gain1/1
  Sum/1 -> Scope/1, Data Type Conversion2/1, Unit Delay1/1
  Abs4/1 -> Discrete PID Controller1/1, Switch/2
  Switch/1 -> Gain4/1
  Gain4/1 -> MATLAB Function2/2(v), MATLAB Function1/2(v)
  MATLAB Function/1(y) -> MATLAB Function1/1(u)
  MATLAB Function/2(x) -> MATLAB Function2/1(u)
  Gain1/1 -> Sum/2
  Gain2/1 -> Sum/1
  Add1/1 -> Error/1

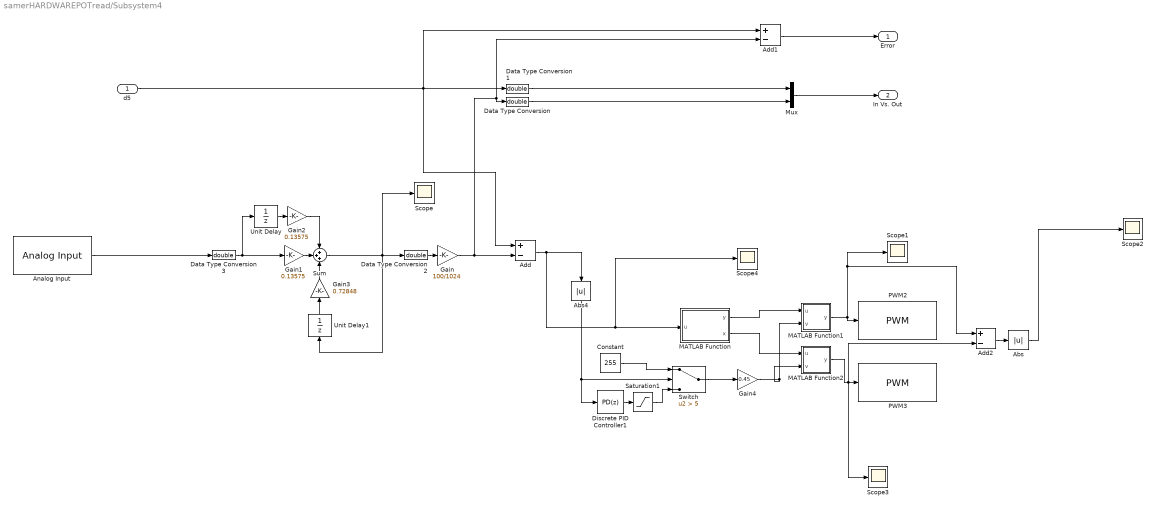
== system samerHARDWAREPOTread/Subsystem4 ==
  d5 : Inport
  Abs : Abs  SaturateOnIntegerOverflow=off
  Abs4 : Abs  SaturateOnIntegerOverflow=off
  Add : Sum  Inputs=+-
  Add1 : Sum  Inputs=+-
  Add2 : Sum  Inputs=+-
  Analog Input : arduinolib/Analog Input  pinNumber=2  ReadResultsOnly=off  ConversionTriggerSource=Software  ExternalTriggerType=uint32( 0 )  OutputDataType=uint16  EnableConversionCompleteNotify=off  EnableOuputStatus=off  SampleTime=0.01  blockPlatform=arduino
  Constant : Constant  Value=255
  Data Type Conversion{,1..3} (4 alike) : DataTypeConversion  OutDataTypeStr=double  SaturateOnIntegerOverflow=off  RndMeth=Floor
  Discrete PID Controller1 : slpidlib/PID Controller  Controller=PD  Form=Parallel  TimeDomain=Discrete-time  UseExternalTs=off  SampleTime=0.01  IntegratorMethod=Forward Euler  FilterMethod=Forward Euler  ControllerParametersSource=internal  P=325  I=3  UseKiTs=off  D=.75  N=1  UseFilter=off  TunerSelectOption=Transfer Function Based (PID Tuner App)  InitialConditionSource=internal  InitialConditionForIntegrator=0  InitialConditionForFilter=0  DifferentiatorICPrevScaledInput=0  ExternalReset=none  TrackingMode=off  Kt=1  LimitOutput=off  SatLimitsSource=internal  UpperSaturationLimit=inf  LowerSaturationLimit=-inf  LinearizeAsGain=off  AntiWindupMode=none  Kb=1  LimitIntegrator=off  UpperIntegratorSaturationLimit=inf  LowerIntegratorSaturationLimit=-inf  POutMin=[]  POutMax=[]  IOutMin=[]  IOutMax=[]  DOutMin=[]  DOutMax=[]  NOutMin=[]  NOutMax=[]  SumOutMin=[]  SumOutMax=[]  SaturationOutMin=[]  SaturationOutMax=[]  PParamMin=[]  PParamMax=[]  IParamMin=[]  IParamMax=[]  DParamMin=[]  DParamMax=[]  NParamMin=[]  NParamMax=[]  KbParamMin=[]  KbParamMax=[]  KtParamMin=[]  KtParamMax=[]  KbOutMin=[]  KbOutMax=[]  KtOutMin=[]  KtOutMax=[]  IntegratorOutMin=[]  IntegratorOutMax=[]  FilterOutMin=[]  FilterOutMax=[]  SumI1OutMin=[]  SumI1OutMax=[]  SumI2OutMin=[]  SumI2OutMax=[]  SumI3OutMin=[]  SumI3OutMax=[]  SumI4OutMin=[]  SumI4OutMax=[]  SumDOutMin=[]  SumDOutMax=[]  DifferentiatorOutMin=[]  DifferentiatorOutMax=[]  FilterDiffOutCoefMin=[]  FilterDiffOutCoefMax=[]  ReciprocalOutMin=[]  ReciprocalOutMax=[]  SumDenOutMin=[]  SumDenOutMax=[]  SumNumOutMin=[]  SumNumOutMax=[]  DivideOutMin=[]  DivideOutMax=[]  UdiffTsProdOutMin=[]  UdiffTsProdOutMax=[]  NTsProdOutMin=[]  NTsProdOutMax=[]  UintegralTsProdOutMin=[]  UintegralTsProdOutMax=[]  UngainTsProdOutMin=[]  UngainTsProdOutMax=[]  ClampingZeroOutDataTypeStr=Inherit: Inherit via back propagation  ClampingZeroOutMin=[]  ClampingZeroOutMax=[]  FilterDenConstantOutDataTypeStr=Inherit: Inherit via back propagation  FilterDenConstantOutMin=[]  FilterDenConstantOutMax=[]  PCopyOutDataTypeStr=Inherit: Inherit via back propagation  PCopyOutMin=[]  PCopyOutMax=[]  NCopyOutDataTypeStr=Inherit: Inherit via back propagation  NCopyOutMin=[]  NCopyOutMax=[]  IntegratorContinuousStateAttributes=''  IntegratorStateMustResolveToSignalObject=off  IntegratorRTWStateStorageClass=Auto  FilterContinuousStateAttributes=''  FilterStateMustResolveToSignalObject=off  FilterRTWStateStorageClass=Auto  ParallelPVariant=InternalParameters  IdealPVariant=Disabled  IVariant=Disabled  DVariant=InternalParameters  IntegratorVariant=Disabled  SatVariant=Disabled  AWVariant=Disabled  PCopyVariant=Disabled  TRVariant=Disabled  FdbkBlocksVariant=Forward  IdealPFdbkVariant=Disabled  SatFdbkVariant=Disabled  DerivativeFilterVariant=Differentiator  NVariant=Passthrough  NCopyVariant=Disabled_SignalSpec  FilterICVariant=InternalICsDifferentiator  IntegratorICVariant=Disabled  ExternalResetVariant=Disabled  TRSumVariant=Passthrough  SumFdbkVariant=Disabled  SumVariant=Sum_PD  TsampFilterVariant=InternalTs  TsampNgainVariant=Passthrough  TsampIntegralVariant=Disabled_SignalSpec  ExternalSaturationOutDataTypeStr=Inherit: Same as second input
      settings: LibrarySourceBlock=simulink/Discrete/Discrete PID Controller
  Gain : Gain  Gain=100/1024
  Gain1 : Gain  Gain=0.13575
  Gain2 : Gain  Gain=0.13575
  Gain3 : Gain  Gain=0.72848
  Gain4 : Gain  Gain=0.45
  MATLAB Function : MATLAB Function  TreatAsAtomicUnit=on
  MATLAB Function1 : MATLAB Function  TreatAsAtomicUnit=on
  MATLAB Function2 : MATLAB Function  TreatAsAtomicUnit=on
  Mux : Mux  Inputs=2
  PWM2 : arduinolib/PWM  pinNumber=8  frequencyType=Default  desiredFrequency=490.2  achievableFrequency=490.2
  PWM3 : arduinolib/PWM  pinNumber=9  frequencyType=Default  desiredFrequency=490.2  achievableFrequency=490.2
  Saturation1 : Saturate  UpperLimit=200  LowerLimit=0
  Scope{,1..4} (5 alike) : Scope
      Scope settings: ActiveDisplayYMinimum=-89.3058  ActiveDisplayYMaximum=803.75221
      Scope1 settings: ActiveDisplayYMinimum=-31.875  ActiveDisplayYMaximum=286.875  DataLoggingVariableName=ScopeData2
      Scope2 settings: DataLoggingVariableName=ScopeData3
      Scope3 settings: ActiveDisplayYMinimum=-31.875  ActiveDisplayYMaximum=286.875  DataLoggingVariableName=ScopeData4
      Scope4 settings: ActiveDisplayYMinimum=-38.33565  ActiveDisplayYMaximum=48.7182
  Sum : Sum  Inputs=+++
  Switch : Switch  Criteria=u2 > Threshold  Threshold=5  SaturateOnIntegerOverflow=off  InputSameDT=off
  Unit Delay : UnitDelay  SampleTime=-1  HasFrameUpgradeWarning=on
  Unit Delay1 : UnitDelay  SampleTime=-1  HasFrameUpgradeWarning=on
  Error : Outport
  In Vs. Out : Outport  Port=2
  wires:
  Unit Delay/1 -> Gain2/1
  Gain3/1 -> Sum/3
  Add2/1 -> Abs/1
  MATLAB Function1/1(y) -> PWM2/1, Add2/1, Scope1/1
  Data Type Conversion2/1 -> Gain/1
  Abs/1 -> Scope2/1
  MATLAB Function2/1(y) -> Scope3/1, Add2/2, PWM3/1
  Add/1 -> Abs4/1, Scope4/1, MATLAB Function/1(u)
  Saturation1/1 -> Switch/3
  Analog Input/1 -> Data Type Conversion3/1
  Unit Delay1/1 -> Gain3/1
  Gain/1 -> Data Type Conversion/1, Add1/2, Add/2
  d5/1 -> Data Type Conversion1/1, Add1/1, Add/1
  Discrete PID Controller1/1 -> Saturation1/1
  Constant/1 -> Switch/1
  Data Type Conversion/1 -> Mux/2
  Data Type Conversion1/1 -> Mux/1
  Mux/1 -> In Vs. Out/1
  Data Type Conversion3/1 -> Unit Delay/1, Gain1/1
  Sum/1 -> Scope/1, Data Type Conversion2/1, Unit Delay1/1
  Abs4/1 -> Discrete PID Controller1/1, Switch/2
  Switch/1 -> Gain4/1
  Gain4/1 -> MATLAB Function2/2(v), MATLAB Function1/2(v)
  MATLAB Function/1(y) -> MATLAB Function1/1(u)
  MATLAB Function/2(x) -> MATLAB Function2/1(u)
  Gain1/1 -> Sum/2
  Gain2/1 -> Sum/1
  Add1/1 -> Error/1

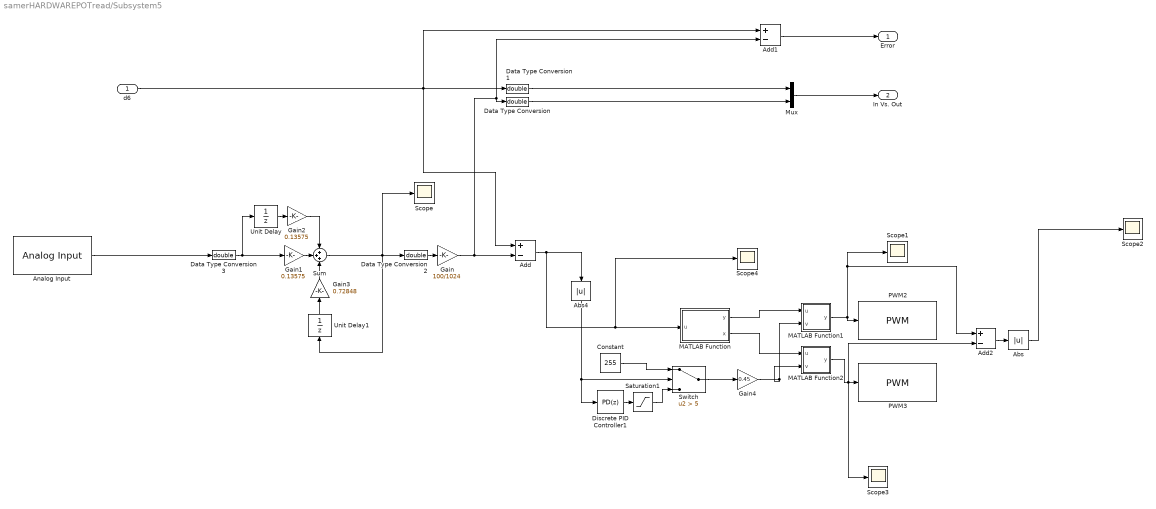
== system samerHARDWAREPOTread/Subsystem5 ==
  d6 : Inport
  Abs : Abs  SaturateOnIntegerOverflow=off
  Abs4 : Abs  SaturateOnIntegerOverflow=off
  Add : Sum  Inputs=+-
  Add1 : Sum  Inputs=+-
  Add2 : Sum  Inputs=+-
  Analog Input : arduinolib/Analog Input  pinNumber=1  ReadResultsOnly=off  ConversionTriggerSource=Software  ExternalTriggerType=uint32( 0 )  OutputDataType=uint16  EnableConversionCompleteNotify=off  EnableOuputStatus=off  SampleTime=0.01  blockPlatform=arduino
  Constant : Constant  Value=255
  Data Type Conversion{,1..3} (4 alike) : DataTypeConversion  OutDataTypeStr=double  SaturateOnIntegerOverflow=off  RndMeth=Floor
  Discrete PID Controller1 : slpidlib/PID Controller  Controller=PD  Form=Parallel  TimeDomain=Discrete-time  UseExternalTs=off  SampleTime=0.01  IntegratorMethod=Forward Euler  FilterMethod=Forward Euler  ControllerParametersSource=internal  P=325  I=3  UseKiTs=off  D=.75  N=1  UseFilter=off  TunerSelectOption=Transfer Function Based (PID Tuner App)  InitialConditionSource=internal  InitialConditionForIntegrator=0  InitialConditionForFilter=0  DifferentiatorICPrevScaledInput=0  ExternalReset=none  TrackingMode=off  Kt=1  LimitOutput=off  SatLimitsSource=internal  UpperSaturationLimit=inf  LowerSaturationLimit=-inf  LinearizeAsGain=off  AntiWindupMode=none  Kb=1  LimitIntegrator=off  UpperIntegratorSaturationLimit=inf  LowerIntegratorSaturationLimit=-inf  POutMin=[]  POutMax=[]  IOutMin=[]  IOutMax=[]  DOutMin=[]  DOutMax=[]  NOutMin=[]  NOutMax=[]  SumOutMin=[]  SumOutMax=[]  SaturationOutMin=[]  SaturationOutMax=[]  PParamMin=[]  PParamMax=[]  IParamMin=[]  IParamMax=[]  DParamMin=[]  DParamMax=[]  NParamMin=[]  NParamMax=[]  KbParamMin=[]  KbParamMax=[]  KtParamMin=[]  KtParamMax=[]  KbOutMin=[]  KbOutMax=[]  KtOutMin=[]  KtOutMax=[]  IntegratorOutMin=[]  IntegratorOutMax=[]  FilterOutMin=[]  FilterOutMax=[]  SumI1OutMin=[]  SumI1OutMax=[]  SumI2OutMin=[]  SumI2OutMax=[]  SumI3OutMin=[]  SumI3OutMax=[]  SumI4OutMin=[]  SumI4OutMax=[]  SumDOutMin=[]  SumDOutMax=[]  DifferentiatorOutMin=[]  DifferentiatorOutMax=[]  FilterDiffOutCoefMin=[]  FilterDiffOutCoefMax=[]  ReciprocalOutMin=[]  ReciprocalOutMax=[]  SumDenOutMin=[]  SumDenOutMax=[]  SumNumOutMin=[]  SumNumOutMax=[]  DivideOutMin=[]  DivideOutMax=[]  UdiffTsProdOutMin=[]  UdiffTsProdOutMax=[]  NTsProdOutMin=[]  NTsProdOutMax=[]  UintegralTsProdOutMin=[]  UintegralTsProdOutMax=[]  UngainTsProdOutMin=[]  UngainTsProdOutMax=[]  ClampingZeroOutDataTypeStr=Inherit: Inherit via back propagation  ClampingZeroOutMin=[]  ClampingZeroOutMax=[]  FilterDenConstantOutDataTypeStr=Inherit: Inherit via back propagation  FilterDenConstantOutMin=[]  FilterDenConstantOutMax=[]  PCopyOutDataTypeStr=Inherit: Inherit via back propagation  PCopyOutMin=[]  PCopyOutMax=[]  NCopyOutDataTypeStr=Inherit: Inherit via back propagation  NCopyOutMin=[]  NCopyOutMax=[]  IntegratorContinuousStateAttributes=''  IntegratorStateMustResolveToSignalObject=off  IntegratorRTWStateStorageClass=Auto  FilterContinuousStateAttributes=''  FilterStateMustResolveToSignalObject=off  FilterRTWStateStorageClass=Auto  ParallelPVariant=InternalParameters  IdealPVariant=Disabled  IVariant=Disabled  DVariant=InternalParameters  IntegratorVariant=Disabled  SatVariant=Disabled  AWVariant=Disabled  PCopyVariant=Disabled  TRVariant=Disabled  FdbkBlocksVariant=Forward  IdealPFdbkVariant=Disabled  SatFdbkVariant=Disabled  DerivativeFilterVariant=Differentiator  NVariant=Passthrough  NCopyVariant=Disabled_SignalSpec  FilterICVariant=InternalICsDifferentiator  IntegratorICVariant=Disabled  ExternalResetVariant=Disabled  TRSumVariant=Passthrough  SumFdbkVariant=Disabled  SumVariant=Sum_PD  TsampFilterVariant=InternalTs  TsampNgainVariant=Passthrough  TsampIntegralVariant=Disabled_SignalSpec  ExternalSaturationOutDataTypeStr=Inherit: Same as second input
      settings: LibrarySourceBlock=simulink/Discrete/Discrete PID Controller
  Gain : Gain  Gain=100/1024
  Gain1 : Gain  Gain=0.13575
  Gain2 : Gain  Gain=0.13575
  Gain3 : Gain  Gain=0.72848
  Gain4 : Gain  Gain=0.45
  MATLAB Function : MATLAB Function  TreatAsAtomicUnit=on
  MATLAB Function1 : MATLAB Function  TreatAsAtomicUnit=on
  MATLAB Function2 : MATLAB Function  TreatAsAtomicUnit=on
  Mux : Mux  Inputs=2
  PWM2 : arduinolib/PWM  pinNumber=6  frequencyType=Default  desiredFrequency=490.2  achievableFrequency=490.2
  PWM3 : arduinolib/PWM  pinNumber=7  frequencyType=Default  desiredFrequency=490.2  achievableFrequency=490.2
  Saturation1 : Saturate  UpperLimit=200  LowerLimit=0
  Scope{,1..4} (5 alike) : Scope
      Scope settings: ActiveDisplayYMinimum=-89.3058  ActiveDisplayYMaximum=803.75221
      Scope1 settings: ActiveDisplayYMinimum=-31.875  ActiveDisplayYMaximum=286.875  DataLoggingVariableName=ScopeData2
      Scope2 settings: DataLoggingVariableName=ScopeData3
      Scope3 settings: ActiveDisplayYMinimum=-31.875  ActiveDisplayYMaximum=286.875  DataLoggingVariableName=ScopeData4
      Scope4 settings: ActiveDisplayYMinimum=-38.33565  ActiveDisplayYMaximum=48.7182
  Sum : Sum  Inputs=+++
  Switch : Switch  Criteria=u2 > Threshold  Threshold=5  SaturateOnIntegerOverflow=off  InputSameDT=off
  Unit Delay : UnitDelay  SampleTime=-1  HasFrameUpgradeWarning=on
  Unit Delay1 : UnitDelay  SampleTime=-1  HasFrameUpgradeWarning=on
  Error : Outport
  In Vs. Out : Outport  Port=2
  wires:
  Unit Delay/1 -> Gain2/1
  Gain3/1 -> Sum/3
  Add2/1 -> Abs/1
  MATLAB Function1/1(y) -> PWM2/1, Add2/1, Scope1/1
  Data Type Conversion2/1 -> Gain/1
  Abs/1 -> Scope2/1
  MATLAB Function2/1(y) -> Scope3/1, Add2/2, PWM3/1
  Add/1 -> Abs4/1, Scope4/1, MATLAB Function/1(u)
  Saturation1/1 -> Switch/3
  Analog Input/1 -> Data Type Conversion3/1
  Unit Delay1/1 -> Gain3/1
  Gain/1 -> Data Type Conversion/1, Add1/2, Add/2
  d6/1 -> Data Type Conversion1/1, Add1/1, Add/1
  Discrete PID Controller1/1 -> Saturation1/1
  Constant/1 -> Switch/1
  Data Type Conversion/1 -> Mux/2
  Data Type Conversion1/1 -> Mux/1
  Mux/1 -> In Vs. Out/1
  Data Type Conversion3/1 -> Unit Delay/1, Gain1/1
  Sum/1 -> Scope/1, Data Type Conversion2/1, Unit Delay1/1
  Abs4/1 -> Discrete PID Controller1/1, Switch/2
  Switch/1 -> Gain4/1
  Gain4/1 -> MATLAB Function2/2(v), MATLAB Function1/2(v)
  MATLAB Function/1(y) -> MATLAB Function1/1(u)
  MATLAB Function/2(x) -> MATLAB Function2/1(u)
  Gain1/1 -> Sum/2
  Gain2/1 -> Sum/1
  Add1/1 -> Error/1

== matlab function samerHARDWAREPOTread/Subsystem3/MATLAB Function1 ==
  data: u input; y output; v input
function y = fcn(u,v)

y = u*v;

== matlab function samerHARDWAREPOTread/Subsystem3/MATLAB Function2 ==
  data: u input; y output; v input
function y = fcn(u,v)

y = u*v;

== matlab function samerHARDWAREPOTread/Subsystem/MATLAB Function ==
  data: u input; y output; x output
function [y,x] = fcn(u)

if u >= 0
    y=1;
    x=0;
else
    y=0;
    x=1;
end

== matlab function samerHARDWAREPOTread/Subsystem4/MATLAB Function ==
  data: u input; y output; x output
function [y,x] = fcn(u)

if u >= 0
    y=1;
    x=0;
else
    y=0;
    x=1;
end

== matlab function samerHARDWAREPOTread/Subsystem4/MATLAB Function1 ==
  data: u input; y output; v input
function y = fcn(u,v)

y = u*v;

== matlab function samerHARDWAREPOTread/Subsystem4/MATLAB Function2 ==
  data: u input; y output; v input
function y = fcn(u,v)

y = u*v;

== matlab function samerHARDWAREPOTread/Subsystem5/MATLAB Function ==
  data: u input; y output; x output
function [y,x] = fcn(u)

if u >= 0
    y=1;
    x=0;
else
    y=0;
    x=1;
end

== matlab function samerHARDWAREPOTread/Subsystem5/MATLAB Function1 ==
  data: u input; y output; v input
function y = fcn(u,v)

y = u*v;

== matlab function samerHARDWAREPOTread/Subsystem5/MATLAB Function2 ==
  data: u input; y output; v input
function y = fcn(u,v)

y = u*v;

== matlab function samerHARDWAREPOTread/MATLAB Function ==
  data: X input; deltaL output; Y input; Z input; Roll input; Pitch input; Yaw input
function deltaL = UPU_IK_Sim(X, Y, Z, Roll, Pitch, Yaw)
%#codegen
% UPU_IK_Sim: Inverse Kinematics for UPU Stewart Platform
%
% Inputs : X, Y, Z         -> translation of platform center [m]
%          Roll, Pitch, Yaw -> rotation angles [rad]
% Output : deltaL(6x1)     -> leg length changes from home [m]
%
% Geometry parameters and base/platform layout defined internally.
% Home length l0 = 0.4 m

%% --- Geometry Definition ---
Rb = 0.185;   % Base radius [m]
Rp = 0.150;  % Platform radius [m]
l0 = 0.29;   % Nominal leg length [m]

% Joint angle layout (hexagonal)
angleB = deg2rad([25 49 145 169 265 289]);
angleP = deg2rad([0 74 120 194 240 314]);

b = zeros(3,6);
p = zeros(3,6);
for i = 1:6
    b(:,i) = [Rb*cos(angleB(i)); Rb*sin(angleB(i)); 0];
    p(:,i) = [Rp*cos(angleP(i)); Rp*sin(angleP(i)); 0];
end

%% --- Desired Pose ---
r = [X; Y; Z]; % translation vector

% Rotation matrix (ZYX order: yaw-pitch-roll)
cy = cos(Yaw); sy = sin(Yaw);
cp = cos(Pitch); sp = sin(Pitch);
cr = cos(Roll); sr = sin(Roll);

R = [cy*cp, cy*sp*sr - sy*cr, cy*sp*cr + sy*sr;
     sy*cp, sy*sp*sr + cy*cr, sy*sp*cr - cy*sr;
     -sp,   cp*sr,            cp*cr];

%% --- Compute Leg Lengths ---
l = zeros(1,6);
for i = 1:6
    L = r + R*p(:,i) - b(:,i);
    l(i) = sqrt(L(1)^2 + L(2)^2 + L(3)^2);
end

%% --- Compute Delta Lengths ---
deltaL = (l - l0)';   % column vector [Δl1..Δl6]
end

== matlab function samerHARDWAREPOTread/Subsystem/MATLAB Function1 ==
  data: u input; y output; v input
function y = fcn(u,v)

y = u*v;

== matlab function samerHARDWAREPOTread/Subsystem/MATLAB Function2 ==
  data: u input; y output; v input
function y = fcn(u,v)

y = u*v;

== matlab function samerHARDWAREPOTread/Subsystem1/MATLAB Function ==
  data: u input; y output; x output
function [y,x] = fcn(u)

if u >= 0
    y=1;
    x=0;
else
    y=0;
    x=1;
end

== matlab function samerHARDWAREPOTread/Subsystem1/MATLAB Function1 ==
  data: u input; y output; v input
function y = fcn(u,v)

y = u*v;

== matlab function samerHARDWAREPOTread/Subsystem1/MATLAB Function2 ==
  data: u input; y output; v input
function y = fcn(u,v)

y = u*v;

== matlab function samerHARDWAREPOTread/Subsystem2/MATLAB Function ==
  data: u input; y output; x output
function [y,x] = fcn(u)

if u >= 0
    y=1;
    x=0;
else
    y=0;
    x=1;
end

== matlab function samerHARDWAREPOTread/Subsystem2/MATLAB Function1 ==
  data: u input; y output; v input
function y = fcn(u,v)

y = u*v;

== matlab function samerHARDWAREPOTread/Subsystem2/MATLAB Function2 ==
  data: u input; y output; v input
function y = fcn(u,v)

y = u*v;

== matlab function samerHARDWAREPOTread/Subsystem3/MATLAB Function ==
  data: u input; y output; x output
function [y,x] = fcn(u)

if u >= 0
    y=1;
    x=0;
else
    y=0;
    x=1;
end
